simulink model "Daolibai_design_SFtu"  (R2016a)
settings: Solver=VariableStepAuto  SolverMode=SingleTasking  StartTime=0.0  StopTime=20  RelTol=1e-3
values from neighbouring files (symbols this model uses):
  A1 = [0 1 0 0 ... (first row only)    [Daolibai_analysis_ControllAndObserv.m]    (also in Daolibai_analysis_stability.m; Daolibai_design_OSF.m; Daolibai_design_OSFandPIOF.m = [A [0 0 0 0]'; Daolibai_design_SF.m)
  B1 = [0;1;0;-2]    [Daolibai_analysis_ControllAndObserv.m]    (also in Daolibai_analysis_stability.m; Daolibai_design_OSF.m; Daolibai_design_OSFandPIOF.m = [B;0]; Daolibai_design_SF.m)
  C1 = [1 0 0 0]    [Daolibai_analysis_ControllAndObserv.m]    (also in Daolibai_analysis_stability.m; Daolibai_design_OSF.m; Daolibai_design_SF.m; Daolibai_design_SFandOF.m)
  K = inv(P1)*V1    [Caishidianlu_design.m]    (also in Daolibai_design_OSF.m = acker(A1,B1,P1); Daolibai_design_OSFandPIOF.m = acker(A1,B1,P); Daolibai_design_SF.m = acker(A1,B1,P); Daolibai_design_SFandOF.m = acker(A,B,P))
settings Model: Creator=19017  LastModifiedBy=19017
settings DataIOCC: ReturnWorkspaceOutputs=on
settings DebuggingCC: SFUnexpectedBacktrackingDiag=error  SFNoUnconditionalDefaultTransitionDiag=error
settings SFSimCC: SimUseLocalCustomCode=on
settings RTWCC: RTWUseLocalCustomCode=on
settings GRTTargetCC: TargetLangStandard=C99 (ISO)
settings ConfigComp: CovMetricSettings=dwe  CovSaveCumulativeToWorkspaceVar=off  CovSaveSingleToWorkspaceVar=off  CovExternalEMLEnable=on

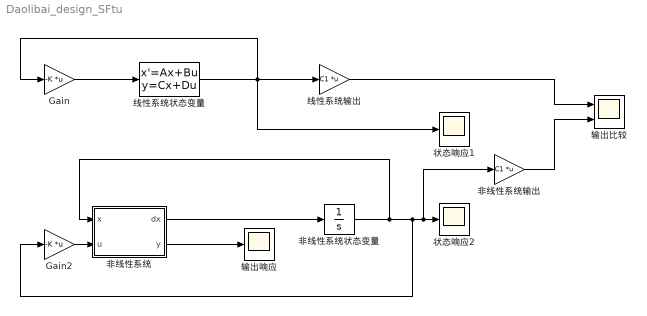
== system Daolibai_design_SFtu ==
  Gain : Gain  Gain=-K  Multiplication=Matrix(K*u)
  Gain2 : Gain  Gain=-K  Multiplication=Matrix(K*u)
  状态响应1 : Scope
  状态响应2 : Scope
  线性系统状态变量 : StateSpace  A=A1  B=B1  C=eye(4)  D=[0;0;0;0]  X0=[0 0 0.01 0.01]
  线性系统输出 : Gain  Gain=C1  Multiplication=Matrix(K*u)
  输出响应 : Scope
  输出比较 : Scope  NumInputPorts=2
  非线性系统 : MATLAB Function  TreatAsAtomicUnit=on
  非线性系统状态变量 : Integrator  InitialCondition=[0 0 0.01 0.01]
  非线性系统输出 : Gain  Gain=C1  Multiplication=Matrix(K*u)
  wires:
  线性系统状态变量/1 -> Gain/1, 线性系统输出/1, 状态响应1/1
  Gain/1 -> 线性系统状态变量/1
  线性系统输出/1 -> 输出比较/1
  非线性系统状态变量/1 -> 非线性系统输出/1, 状态响应2/1, Gain2/1, 非线性系统/1(x)
  Gain2/1 -> 非线性系统/2(u)
  非线性系统/2(y) -> 输出响应/1
  非线性系统输出/1 -> 输出比较/2
  非线性系统/1(dx) -> 非线性系统状态变量/1

== matlab function Daolibai_design_SFtu/非线性系统 ==
  data: dx output; x input; u input; y output
function [dx,y] = fcn(x,u)
dx = zeros(4,1);
M = 1;
m = 0.1;
l = 0.5;
g = 9.8;
dx(1) = x(2);
dx(2) = (u+m*l*x(4)^2*sin(x(3))-m*g*sin(x(3))*cos(x(3)))/(M+m-m*cos(x(3))^2);
dx(3) = x(4);
dx(4) = (-u*cos(x(3))+(M+m)*g*sin(x(3))-m*l*x(4)^2*sin(x(3))*cos(x(3)))/((M+m)*l-m*l*cos(x(3))^2);
y = x(1);
